simulink model "test"  (R2016b)
settings: Solver=FixedStepAuto  StartTime=0.0  StopTime=12.0  FixedStep=1e-3  RelTol=1e-3
undefined symbols (not defined in the file or in its folder): MultiQ, PCI, Quanser
libraries: sldrtlib x3
settings Model: SimulationMode=external  Creator=Labos1  LastModifiedBy=Labos1
settings RTWCC: SystemTargetFile=sldrt.tlc  TemplateMakefile=sldrt.tmf  Description=Simulink Desktop Real-Time  RTWCompilerOptimization=on
settings CodeAppCC: MaxIdLength=95
settings SimulinkDesktopRealTimeCC: TargetPreCompLibLocation=C:\Program Files\MATLAB\R2016b\toolbox\sldrt\lib\win64  SupportVariableSizeSignals=off

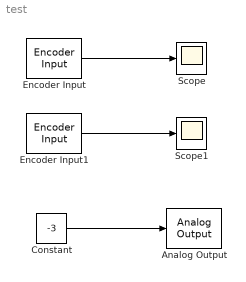
== system test ==
  Analog Output : sldrtlib/Analog Output  SampleTime=1e-3  MaxMissedTicks=10  ShowMissedTicks=off  YieldWhenWaiting=off  DrvName=Quanser/MultiQ-PCI  DrvAddress=4294967295  DrvOptions=zeros(1,0)  Channels=1  RangeMode=1  VoltRange=1  InitialValue=0  FinalValue=0
      settings: AttributesFormatString=Quanser\nMultiQ-PCI [auto]
  Constant : Constant  Value=-3
  Encoder Input : sldrtlib/Encoder Input  SampleTime=1e-3  MaxMissedTicks=10  ShowMissedTicks=off  YieldWhenWaiting=off  DrvName=Quanser/MultiQ-PCI  DrvAddress=4294967295  DrvOptions=zeros(1,0)  Channels=1  QuadMode=3  IndexPulse=2  InputFilter=Inf  DataType=1
      settings: AttributesFormatString=Quanser\nMultiQ-PCI [auto]
  Encoder Input1 : sldrtlib/Encoder Input  SampleTime=1e-3  MaxMissedTicks=10  ShowMissedTicks=off  YieldWhenWaiting=off  DrvName=Quanser/MultiQ-PCI  DrvAddress=4294967295  DrvOptions=zeros(1,0)  Channels=2  QuadMode=3  IndexPulse=2  InputFilter=Inf  DataType=1
      settings: AttributesFormatString=Quanser\nMultiQ-PCI [auto]
  Scope : Scope
  Scope1 : Scope
  wires:
  Encoder Input/1 -> Scope/1
  Encoder Input1/1 -> Scope1/1
  Constant/1 -> Analog Output/1
